simulink model "final_prj"  (R2018a)
settings: Solver=ode4  StartTime=0.0  StopTime=10.0  FixedStep=0.05  RelTol=1e-3
undefined symbols (not defined in the file or in its folder): DiscIntNeverNeededParam
libraries: fuzblock x6, simulink x2
settings Model: Creator=Mertcan  LastModifiedBy=Mertcan

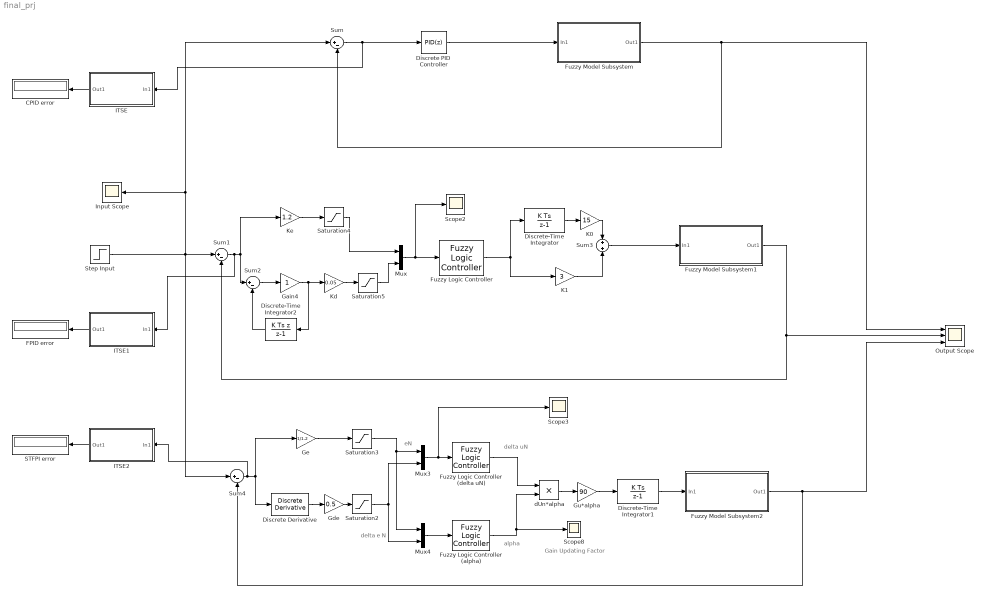
== system final_prj ==
  note: Gain Updating Factor
  note: delta uN
  note: delta e N
  note: eN
  note: alpha
  CPID error : Display
  Discrete Derivative : simulink/Quick Insert/Discrete/Discrete Derivative  gainval=1.0  ICPrevScaledInput=0.0  OutMin=[]  OutMax=[]  OutDataType=fixdt(1, 16)  OutScaling=2^-10  DoSatur=off
      settings: SourceProductName=Simulink  SourceProductBaseCode=SL
  Discrete PID Controller : simulink/Continuous/PID Controller  Controller=PID  TimeDomain=Discrete-time  SampleTime=-1  IntegratorMethod=Forward Euler  FilterMethod=Forward Euler  Form=Parallel  UseFilter=on  ControllerParametersSource=internal  P=1  I=30  D=2  N=1  InitialConditionSource=internal  InitialConditionForIntegrator=0  InitialConditionForFilter=0  ExternalReset=none  LimitOutput=off  UpperSaturationLimit=inf  LowerSaturationLimit=-inf  LinearizeAsGain=off  AntiWindupMode=none  Kb=1  TrackingMode=off  Kt=1  PParamMin=[]  PParamMax=[]  IParamMin=[]  IParamMax=[]  DParamMin=[]  DParamMax=[]  NParamMin=[]  NParamMax=[]  KbParamMin=[]  KbParamMax=[]  KtParamMin=[]  KtParamMax=[]  POutMin=[]  POutMax=[]  IOutMin=[]  IOutMax=[]  DOutMin=[]  DOutMax=[]  NOutMin=[]  NOutMax=[]  KbOutMin=[]  KbOutMax=[]  KtOutMin=[]  KtOutMax=[]  IntegratorOutMin=[]  IntegratorOutMax=[]  FilterOutMin=[]  FilterOutMax=[]  SumOutMin=[]  SumOutMax=[]  SumI1OutMin=[]  SumI1OutMax=[]  SumI2OutMin=[]  SumI2OutMax=[]  SumI3OutMin=[]  SumI3OutMax=[]  SumDOutMin=[]  SumDOutMax=[]  SaturationOutMin=[]  SaturationOutMax=[]  IntegratorContinuousStateAttributes=''  IntegratorStateMustResolveToSignalObject=off  IntegratorRTWStateStorageClass=Auto  FilterContinuousStateAttributes=''  FilterStateMustResolveToSignalObject=off  FilterRTWStateStorageClass=Auto  DifferentiatorICPrevScaledInput=0  DifferentiatorOutMin=[]  DifferentiatorOutMax=[]  FilterDiffOutCoefMin=[]  FilterDiffOutCoefMax=[]  SumDenOutMin=[]  SumDenOutMax=[]  SumNumOutMin=[]  SumNumOutMax=[]  ReciprocalOutMin=[]  ReciprocalOutMax=[]  DivideOutMin=[]  DivideOutMax=[]  TunerSelectOption=Transfer Function Based (PID Tuner App)
  Discrete-Time Integrator : DiscreteIntegrator  SampleTime=-1  ICPrevOutput=DiscIntNeverNeededParam  ICPrevScaledInput=DiscIntNeverNeededParam
  Discrete-Time Integrator1 : DiscreteIntegrator  SampleTime=-1  ICPrevOutput=DiscIntNeverNeededParam  ICPrevScaledInput=DiscIntNeverNeededParam
  Discrete-Time Integrator2 : DiscreteIntegrator  IntegratorMethod=Integration: Backward Euler  SampleTime=-1  ICPrevOutput=DiscIntNeverNeededParam  ICPrevScaledInput=DiscIntNeverNeededParam
  FPID error : Display
  Fuzzy Logic Controller : fuzblock/Fuzzy Logic  Controller  FIS='controller.fis'  OutputSampleNumber=101  DataType=double  FuzzifiedInputs=off  RuleFiringStrengths=off  RuleOutputs=off  AggregatedOutputs=off  SimulateUsing=Interpreted execution  OutOfRangeInputValueMessage=warning  NoRuleFiredMessage=warning  EmptyOutputFuzzySetMessage=warning
  Fuzzy Logic Controller (delta uN) : fuzblock/Fuzzy Logic  Controller  FIS='controller.fis'  OutputSampleNumber=101  DataType=double  FuzzifiedInputs=off  RuleFiringStrengths=off  RuleOutputs=off  AggregatedOutputs=off  SimulateUsing=Interpreted execution  OutOfRangeInputValueMessage=warning  NoRuleFiredMessage=warning  EmptyOutputFuzzySetMessage=warning
  Fuzzy Logic Controller (alpha) : fuzblock/Fuzzy Logic  Controller  FIS='alpha.fis'  OutputSampleNumber=101  DataType=double  FuzzifiedInputs=off  RuleFiringStrengths=off  RuleOutputs=off  AggregatedOutputs=off  SimulateUsing=Interpreted execution  OutOfRangeInputValueMessage=warning  NoRuleFiredMessage=warning  EmptyOutputFuzzySetMessage=warning
  Fuzzy Model Subsystem : Subsystem
  Fuzzy Model Subsystem1 : Subsystem
  Fuzzy Model Subsystem2 : Subsystem
  Gain4 : Gain
  Gde : Gain  Gain=0.5
  Ge : Gain  Gain=1/1.2
  Gu*alpha : Gain  Gain=90
  ITSE : Subsystem
  ITSE1 : Subsystem
  ITSE2 : Subsystem
  Input Scope : Scope
  K0 : Gain  Gain=15
  K1 : Gain  Gain=3
  Kd : Gain  Gain=0.05
  Ke : Gain  Gain=1.2
  Mux : Mux  Inputs=2
  Mux3 : Mux  Inputs=2
  Mux4 : Mux  Inputs=2
  Output Scope : Scope  NumInputPorts=3
  STFPI error : Display
  Saturation{2..5} (4 alike) : Saturate  UpperLimit=1  LowerLimit=-1
  Scope2 : Scope
  Scope3 : Scope
  Scope8 : Scope
  Step Input : Step  Time=0  After=0.6  SampleTime=0
  Sum{,1..2,4} (4 alike) : Sum  Inputs=|+-
  Sum3 : Sum
  dUn*alpha : Product
  wires:
  Fuzzy Model Subsystem/1(Out1) -> Sum/2, Output Scope/1
  Discrete PID Controller/1 -> Fuzzy Model Subsystem/1(In1)
  Fuzzy Model Subsystem1/1(Out1) -> Sum1/2, Output Scope/2
  Sum2/1 -> Gain4/1
  Discrete-Time Integrator2/1 -> Sum2/2
  Gain4/1 -> Discrete-Time Integrator2/1, Kd/1
  Discrete-Time Integrator/1 -> K0/1
  Fuzzy Logic Controller/1 -> K1/1, Discrete-Time Integrator/1
  K1/1 -> Sum3/2
  K0/1 -> Sum3/1
  Mux/1 -> Scope2/1, Fuzzy Logic Controller/1
  Ke/1 -> Saturation4/1
  Fuzzy Model Subsystem2/1(Out1) -> Output Scope/3, Sum4/2
  Fuzzy Logic Controller (delta uN)/1 -> dUn*alpha/1
  Ge/1 -> Saturation3/1
  dUn*alpha/1 -> Gu*alpha/1
  Fuzzy Logic Controller (alpha)/1 -> dUn*alpha/2, Scope8/1
  Mux4/1 -> Fuzzy Logic Controller (alpha)/1
  Mux3/1 -> Scope3/1, Fuzzy Logic Controller (delta uN)/1
  Gde/1 -> Saturation2/1
  Saturation3/1 -> Mux4/1, Mux3/1
  Saturation2/1 -> Mux4/2, Mux3/2
  Sum/1 -> ITSE/1(In1), Discrete PID Controller/1
  ITSE/1(Out1) -> CPID error/1
  ITSE1/1(Out1) -> FPID error/1
  Sum1/1 -> ITSE1/1(In1), Sum2/1, Ke/1
  Sum3/1 -> Fuzzy Model Subsystem1/1(In1)
  Gu*alpha/1 -> Discrete-Time Integrator1/1
  Sum4/1 -> ITSE2/1(In1), Discrete Derivative/1, Ge/1
  ITSE2/1(Out1) -> STFPI error/1
  Saturation4/1 -> Mux/1
  Kd/1 -> Saturation5/1
  Saturation5/1 -> Mux/2
  Step Input/1 -> Sum1/1, Sum4/1, Sum/1, Input Scope/1
  Discrete Derivative/1 -> Gde/1
  Discrete-Time Integrator1/1 -> Fuzzy Model Subsystem2/1(In1)

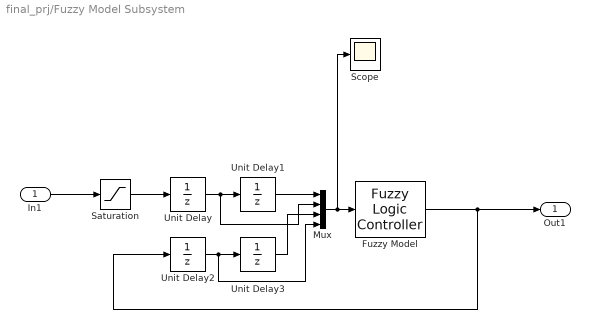
== system final_prj/Fuzzy Model Subsystem ==
  In1 : Inport
  Fuzzy Model : fuzblock/Fuzzy Logic  Controller  FIS='model_narx.fis'  OutputSampleNumber=101  DataType=double  FuzzifiedInputs=off  RuleFiringStrengths=off  RuleOutputs=off  AggregatedOutputs=off  SimulateUsing=Interpreted execution  OutOfRangeInputValueMessage=warning  NoRuleFiredMessage=warning  EmptyOutputFuzzySetMessage=warning
  Mux : Mux
  Saturation : Saturate  UpperLimit=6  LowerLimit=0
  Scope : Scope
  Unit Delay{,1..3} (4 alike) : UnitDelay  SampleTime=-1
  Out1 : Outport
  wires:
  Mux/1 -> Scope/1, Fuzzy Model/1
  Unit Delay2/1 -> Unit Delay3/1, Mux/4
  Fuzzy Model/1 -> Out1/1, Unit Delay2/1
  Unit Delay/1 -> Mux/2, Unit Delay1/1
  Unit Delay1/1 -> Mux/1
  Unit Delay3/1 -> Mux/3
  In1/1 -> Saturation/1
  Saturation/1 -> Unit Delay/1

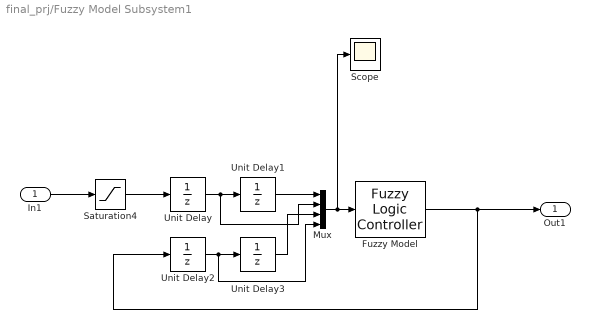
== system final_prj/Fuzzy Model Subsystem1 ==
  In1 : Inport
  Fuzzy Model : fuzblock/Fuzzy Logic  Controller  FIS='model_narx.fis'  OutputSampleNumber=101  DataType=double  FuzzifiedInputs=off  RuleFiringStrengths=off  RuleOutputs=off  AggregatedOutputs=off  SimulateUsing=Interpreted execution  OutOfRangeInputValueMessage=warning  NoRuleFiredMessage=warning  EmptyOutputFuzzySetMessage=warning
  Mux : Mux
  Saturation4 : Saturate  UpperLimit=6  LowerLimit=0
  Scope : Scope
  Unit Delay{,1..3} (4 alike) : UnitDelay  SampleTime=-1
  Out1 : Outport
  wires:
  Mux/1 -> Scope/1, Fuzzy Model/1
  Unit Delay2/1 -> Unit Delay3/1, Mux/4
  Fuzzy Model/1 -> Out1/1, Unit Delay2/1
  Unit Delay/1 -> Mux/2, Unit Delay1/1
  Unit Delay1/1 -> Mux/1
  Unit Delay3/1 -> Mux/3
  In1/1 -> Saturation4/1
  Saturation4/1 -> Unit Delay/1

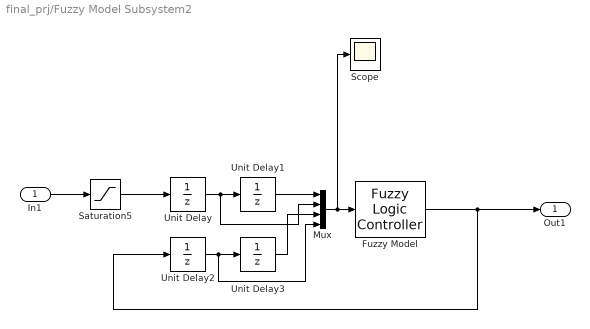
== system final_prj/Fuzzy Model Subsystem2 ==
  In1 : Inport
  Fuzzy Model : fuzblock/Fuzzy Logic  Controller  FIS='model_narx.fis'  OutputSampleNumber=101  DataType=double  FuzzifiedInputs=off  RuleFiringStrengths=off  RuleOutputs=off  AggregatedOutputs=off  SimulateUsing=Interpreted execution  OutOfRangeInputValueMessage=warning  NoRuleFiredMessage=warning  EmptyOutputFuzzySetMessage=warning
  Mux : Mux
  Saturation5 : Saturate  UpperLimit=6  LowerLimit=0
  Scope : Scope
  Unit Delay{,1..3} (4 alike) : UnitDelay  SampleTime=-1
  Out1 : Outport
  wires:
  Mux/1 -> Scope/1, Fuzzy Model/1
  Unit Delay2/1 -> Unit Delay3/1, Mux/4
  Fuzzy Model/1 -> Out1/1, Unit Delay2/1
  Unit Delay/1 -> Mux/2, Unit Delay1/1
  Unit Delay1/1 -> Mux/1
  Unit Delay3/1 -> Mux/3
  In1/1 -> Saturation5/1
  Saturation5/1 -> Unit Delay/1

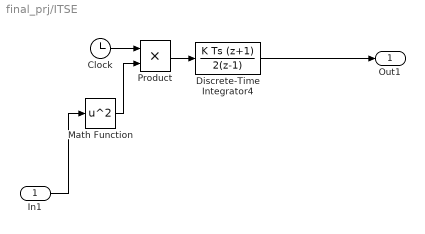
== system final_prj/ITSE ==
  In1 : Inport
  Clock : Clock
  Discrete-Time Integrator4 : DiscreteIntegrator  IntegratorMethod=Integration: Trapezoidal  SampleTime=-1  ICPrevOutput=DiscIntNeverNeededParam  ICPrevScaledInput=DiscIntNeverNeededParam
  Math Function : Math  Operator=square  SaturateOnIntegerOverflow=on
  Product : Product
  Out1 : Outport
  wires:
  Product/1 -> Discrete-Time Integrator4/1
  Clock/1 -> Product/1
  Discrete-Time Integrator4/1 -> Out1/1
  Math Function/1 -> Product/2
  In1/1 -> Math Function/1

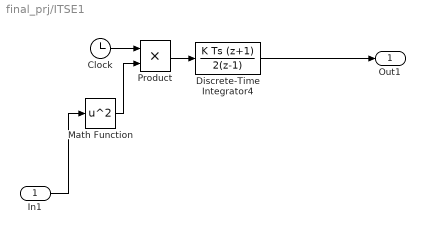
== system final_prj/ITSE1 ==
  In1 : Inport
  Clock : Clock
  Discrete-Time Integrator4 : DiscreteIntegrator  IntegratorMethod=Integration: Trapezoidal  SampleTime=-1  ICPrevOutput=DiscIntNeverNeededParam  ICPrevScaledInput=DiscIntNeverNeededParam
  Math Function : Math  Operator=square  SaturateOnIntegerOverflow=on
  Product : Product
  Out1 : Outport
  wires:
  Product/1 -> Discrete-Time Integrator4/1
  Clock/1 -> Product/1
  Discrete-Time Integrator4/1 -> Out1/1
  Math Function/1 -> Product/2
  In1/1 -> Math Function/1

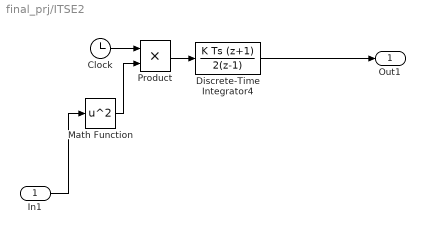
== system final_prj/ITSE2 ==
  In1 : Inport
  Clock : Clock
  Discrete-Time Integrator4 : DiscreteIntegrator  IntegratorMethod=Integration: Trapezoidal  SampleTime=-1  ICPrevOutput=DiscIntNeverNeededParam  ICPrevScaledInput=DiscIntNeverNeededParam
  Math Function : Math  Operator=square  SaturateOnIntegerOverflow=on
  Product : Product
  Out1 : Outport
  wires:
  Product/1 -> Discrete-Time Integrator4/1
  Clock/1 -> Product/1
  Discrete-Time Integrator4/1 -> Out1/1
  Math Function/1 -> Product/2
  In1/1 -> Math Function/1
